simulink model "ipc_ut"  (Simulink 8.1)
settings: Solver=FixedStepDiscrete  StartTime=0.0  StopTime=Inf  FixedStep=0.005  RelTol=1e-3
PostLoadFcn:
  | , if any(exist('dsrtsu_mdlpostloadfcn', 'file') == [2, 3, 6]), try dsrtsu_mdlpostloadfcn('Execute', bdroot); catch fprintf('Error in PostLoadFcn (dsrtsu_mdlpostloadfcn) for model "%s":\n %s\n', bdroot, lasterr); end, end,
libraries: siltestlib x7, idiada_lib x6, ipc x1
settings Model: DSRTSU_INTERNAL_RTI_VER=450  DSRTSU_INTERNAL_RTI_TYPE=rti1401  RTICANMMDATA=struct('GeneralSetupData',struct('modelroot','D:\ELN150201_TAIWAN\trunk\AdasDragon\software\sw_development\arch\app\ifo','generalsettings',struct('filesettings',struct('destfolder',struct('Name','RTICANMM_FILES','Check',1),'buildfolder',struct('Name','.','Check',1),'AbsDestfolder',struct('Name','D:\ELN150201_TAIWAN\trunk\AdasDragon\software\sw_development\arch\app\ifo\RTICANMM_FILES'),'AbsBuildfolder',struct('Name','D:\ELN150201_TAIWAN\trunk\AdasDragon\software\sw_development\arch\app\ifo'))),'options',struct('addpaths',1,'rmpaths',1,'addtrcexclusion',logical(1),'cannavigator',struct('checkmonitoring',0),'show_usrtrc',0,'use_usrtrc',0),'advanced',struct('options',[1 1 1 1 1 1 1 1 1 1 1 1 1 1 1 1 1 1 1 1 1 1 1 1 1 1 1 1 1 1 1 1 1 1 1 1 1 1 1 1 1 1 1 1 1 1 1 1 1 1 1 1 1 1 1 1 1 1 1 1 1 1 1 1 1 1 1 1 1 1 1 1 1 1 1 1 1 1 1 1 1 1 1 1 1 1 1 1 1 1 1 1 1 1 1 1 1 1 1 1]),'MPSetup',{{}},'modelname','ipc_ut','block','ipc_ut'))  DSRTSU_INTERNAL_RTIFPGA=40  Creator=tescamilla  LastModifiedBy=AT015555  BufferReuse=off
settings DataIOCC: SignalLoggingSaveFormat=Dataset
settings OptimizationCC: BlockReduction=off  OptimizeBlockIOStorage=off  BufferReuse=off  ExpressionFolding=off  ExpressionDepthLimit=128  LocalBlockOutputs=off
settings DebuggingCC: FcnCallInpInsideContextMsg=EnableAllAsError
settings HardwareCC: ProdIntDivRoundTo=Zero  ProdEndianess=BigEndian  ProdHWDeviceType=Generic->Custom  TargetIntDivRoundTo=Zero  TargetEndianess=BigEndian  TargetHWDeviceType=Generic->Custom
settings RTWCC: SystemTargetFile=rti1401.tlc  MakeCommand=make_rti  TemplateMakefile=rti1401.tmf  Description=dSPACE DS1401 Hardware Platform  ProcessScript=rti1401_make_rtw_hook
settings STFCustomTargetCC: CodeReplacementLibrary=ANSI_C  ParMdlRefBuildCompliant=on  GeneratePreprocessorConditionals=Disable all  MatFileLogging=on  SystemTargetFile=rti1401.tlc
settings GRTTargetCC: CompOptLevelCompliant=off  ConcurrentExecutionCompliant=off  ExtModeMexFile=noextcomm
settings CustomProperty: DataType=RTWOptions_EnumType_C__Program Files (x86)_dSPACE RCPHIL 2014-B_MATLAB_RTI_RTI1401_TLC_rti1401_1InitialSimState  Value=RUN
settings EnumStrPairs: String=RUN

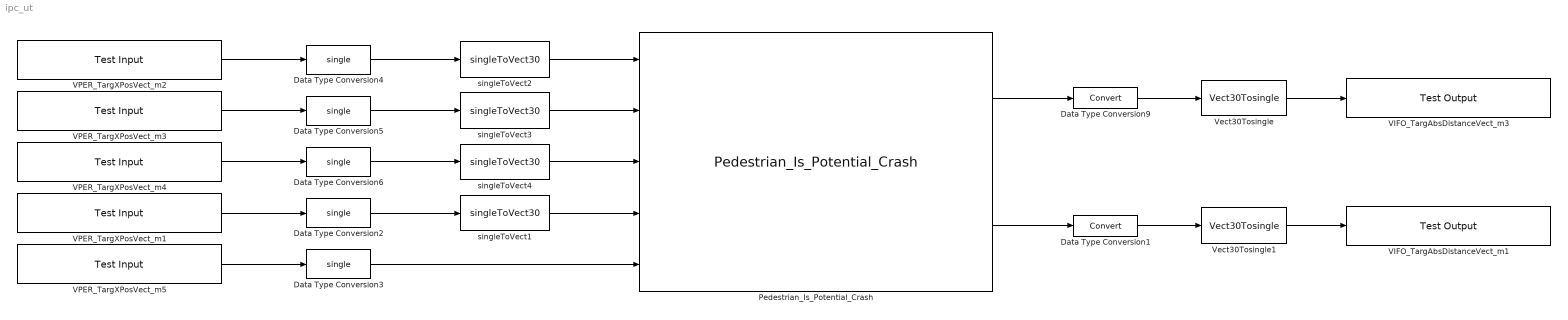
== system ipc_ut ==
  Data Type Conversion1 : DataTypeConversion
  Data Type Conversion{2..6} (5 alike) : DataTypeConversion  OutDataTypeStr=single
  Data Type Conversion9 : DataTypeConversion
  Pedestrian_Is_Potential_Crash : ipc/Pedestrian_Is_Potential_Crash
  VIFO_TargAbsDistanceVect_m1 : siltestlib/Test Output  varname=VIFO_PossibleCrashVect30_flg  sampletime=-1
  VIFO_TargAbsDistanceVect_m3 : siltestlib/Test Output  varname=VIFO_SimpleTTCxVect30_s  sampletime=-1
  VPER_TargXPosVect_m1 : siltestlib/Test Input  varname=VIFO_TargRelSpeedXVect30_mps  sampletime=0.005
  VPER_TargXPosVect_m2 : siltestlib/Test Input  varname=VPER_TargYPosVect30_m  sampletime=0.005
  VPER_TargXPosVect_m3 : siltestlib/Test Input  varname=VIFO_TargAbsSpeedYVect30_mps  sampletime=0.005
  VPER_TargXPosVect_m4 : siltestlib/Test Input  varname=VPER_TargXPosVect30_m  sampletime=0.005
  VPER_TargXPosVect_m5 : siltestlib/Test Input  varname=VIFO_LateralPosition_m  sampletime=0.005
  Vect30Tosingle : idiada_lib/Vect30Tosingle
  Vect30Tosingle1 : idiada_lib/Vect30Tosingle
  singleToVect{1..4} (4 alike) : idiada_lib/singleToVect30
  wires:
  VPER_TargXPosVect_m2/1 -> Data Type Conversion4/1
  Data Type Conversion4/1 -> singleToVect2/1
  VPER_TargXPosVect_m3/1 -> Data Type Conversion5/1
  Data Type Conversion5/1 -> singleToVect3/1
  VPER_TargXPosVect_m4/1 -> Data Type Conversion6/1
  Data Type Conversion6/1 -> singleToVect4/1
  singleToVect3/1 -> Pedestrian_Is_Potential_Crash/2
  singleToVect2/1 -> Pedestrian_Is_Potential_Crash/1
  singleToVect4/1 -> Pedestrian_Is_Potential_Crash/3
  Data Type Conversion9/1 -> Vect30Tosingle/1
  Pedestrian_Is_Potential_Crash/1 -> Data Type Conversion9/1
  Vect30Tosingle/1 -> VIFO_TargAbsDistanceVect_m3/1
  Data Type Conversion1/1 -> Vect30Tosingle1/1
  Vect30Tosingle1/1 -> VIFO_TargAbsDistanceVect_m1/1
  Pedestrian_Is_Potential_Crash/2 -> Data Type Conversion1/1
  VPER_TargXPosVect_m1/1 -> Data Type Conversion2/1
  Data Type Conversion2/1 -> singleToVect1/1
  singleToVect1/1 -> Pedestrian_Is_Potential_Crash/4
  VPER_TargXPosVect_m5/1 -> Data Type Conversion3/1
  Data Type Conversion3/1 -> Pedestrian_Is_Potential_Crash/5
